simulink model "Supply_Chain_II"  (R2018b)
settings: Solver=VariableStepAuto  StartTime=0.0  StopTime=n_T  RelTol=1e-3
undefined symbols (not defined in the file or in its folder): D, m, MTBF_h, n, yoi
libraries: simulink x6
settings Model: Creator=Jorrit de Jong  LastModifiedBy=Jorrit de Jong

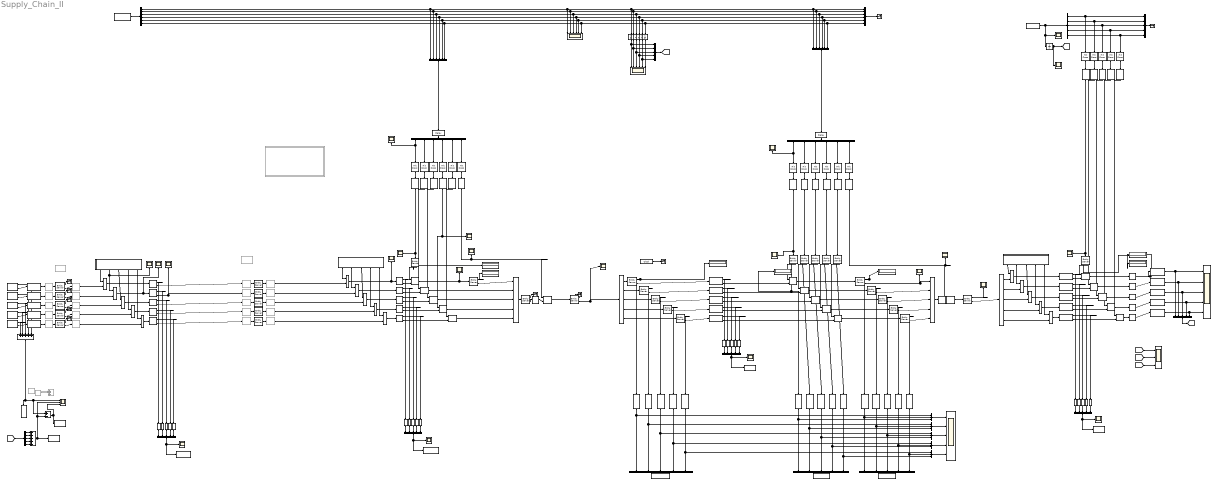
== system Supply_Chain_II ==
  note: DC
  note: Performance measurement JIT
  note: Local warehouse
  note: Island
  note: Performance measurement
  note: Terminal
  note: Performance measurement
  note: Control agent
  note: Performance measurement
  note: Control agent
  note: Source
  note: Performance measurement
  note: Scopes
  note: Nr of parts departed
  Add : Sum  Inputs=+++++
  Add1 : Sum  Inputs=+++++
  Add2 : Sum  Inputs=+-
  Add3 : Sum  Commented=on  Inputs=+++
  Arrived spares : Display
  Blade terminator : EntityTerminator  InputPortMessageModes=m  NumberEntitiesArrived=on
      settings: OutputPortMap=o0
  C terminator : EntityTerminator  InputPortMessageModes=m  NumberEntitiesArrived=on
      settings: OutputPortMap=o0
  Components arrived : Scope  NumInputPorts=5
  Constant : Constant  Commented=on  Value=5*20
  Constant1 : Constant  Commented=on  Value=5*20
  Counter : EntityServer  InputPortMessageModes=m  OutputPortMessageModes=n,m  Capacity=inf  ServiceTimeValue=0  NumberEntitiesDeparted=on
      settings: OutputPortMap=o0,o9
  Counter2 : EntityServer  InputPortMessageModes=m  OutputPortMessageModes=n,m  Capacity=inf  ServiceTimeValue=0  NumberEntitiesDeparted=on
      settings: OutputPortMap=o0,o9
  D terminator : EntityTerminator  InputPortMessageModes=m  NumberEntitiesArrived=on
      settings: OutputPortMap=o0
  DC transport signal : Scope
  DC trigger : Scope
  DC trigger system : Subsystem  Commented=on
  DC trigger1 : Scope
  Data Type Conversion{,1..39} (40 alike) : DataTypeConversion
  Demand - delivery flow : Scope  NumInputPorts=3
  Demux : Demux  Outputs=6
  Demux1 : Demux  Outputs=5
  Demux2 : Demux  Outputs=5
  Demux3 : Demux  Outputs=6
  Demux5 : Demux  Outputs=6
  Departed/Arrived components : Scope  NumInputPorts=3
  Digital Clock : DigitalClock
  Display : Display
  Display1 : Display
  Display2 : Display
  E terminator : EntityTerminator  InputPortMessageModes=m  NumberEntitiesArrived=on
      settings: OutputPortMap=o0
  Entity Input Switch : EntityInputSwitch  InputPortMessageModes=m,m,m,m,m  OutputPortMessageModes=m  NumberInputPorts=5
      settings: InputPortMap=u1,u2,u3,u4,u5
  Entity Input Switch{1..5,7..16} (15 alike) : EntityInputSwitch  InputPortMessageModes=m,m  OutputPortMessageModes=m
  Entity Input Switch6 : EntityInputSwitch  InputPortMessageModes=m,m,m,m,m  OutputPortMessageModes=m  NumberInputPorts=5
      settings: InputPortMap=u1,u2,u3,u4,u5
  Entity Output Switch : EntityOutputSwitch  InputPortMessageModes=m  OutputPortMessageModes=m,m,m,m,m  NumberOutputPorts=5  SwitchingCriterion=From attribute  SwitchAttributeName=PartNumber
      settings: OutputPortMap=o0,o1,o2,o3,o4
  Entity Output Switch1 : EntityOutputSwitch  InputPortMessageModes=m  OutputPortMessageModes=m,m,m,m,m  NumberOutputPorts=5  SwitchingCriterion=From attribute  SwitchAttributeName=PartNumber
      settings: OutputPortMap=o0,o1,o2,o3,o4
  Entity Gate{,1..16} (17 alike) : EntityGate  InputPortMessageModes=m,m  OutputPortMessageModes=m  OperatingMode=Release gate
  Entity Generator : EntityGenerator  OutputPortMessageModes=n,m  Period=MTBF_h(1,yoi)  GenerateEntityAtSimulationStart=off  AttributeName=PartNumber  NumberEntitiesDeparted=on  EntityType=Structured  EntityTypeName=Part
      settings: OutputPortMap=o0,o3
  Entity Generator1 : EntityGenerator  OutputPortMessageModes=n,m  Period=MTBF_h(2,yoi)  GenerateEntityAtSimulationStart=off  AttributeName=PartNumber  AttributeInitialValue=2  NumberEntitiesDeparted=on  EntityType=Structured  EntityTypeName=Part
      settings: OutputPortMap=o0,o3
  Entity Generator{5..16,18..22} (17 alike) : EntityGenerator  InputPortMessageModes=m  OutputPortMessageModes=m  GenerationMethod=Event-based  AttributeName=entity  AttributeInitialValue=0  EntityTypeName=Entity
      settings: InputPortMap=u0
  Entity Generator2 : EntityGenerator  OutputPortMessageModes=n,m  Period=MTBF_h(3,yoi)  GenerateEntityAtSimulationStart=off  AttributeName=PartNumber  AttributeInitialValue=3  NumberEntitiesDeparted=on  EntityType=Structured  EntityTypeName=Part
      settings: OutputPortMap=o0,o3
  Entity Generator3 : EntityGenerator  OutputPortMessageModes=n,m  Period=MTBF_h(4,yoi)  GenerateEntityAtSimulationStart=off  AttributeName=PartNumber  AttributeInitialValue=4  NumberEntitiesDeparted=on  EntityType=Structured  EntityTypeName=Part
      settings: OutputPortMap=o0,o3
  Entity Generator4 : EntityGenerator  OutputPortMessageModes=n,m  Period=MTBF_h(5,yoi)  GenerateEntityAtSimulationStart=off  AttributeName=PartNumber  AttributeInitialValue=5  NumberEntitiesDeparted=on  EntityType=Structured  EntityTypeName=Part
      settings: OutputPortMap=o0,o3
  Entity Queue{,1..4} (5 alike) : EntityQueue  InputPortMessageModes=m  OutputPortMessageModes=n,m  Capacity=20  NumberEntitiesInBlock=on
      settings: OutputPortMap=o1,o5
  Entity Queue{10..14} (5 alike) : EntityQueue  InputPortMessageModes=m  OutputPortMessageModes=m
      settings: OutputPortMap=o5
  Entity Queue{5..9} (5 alike) : EntityQueue  InputPortMessageModes=m  OutputPortMessageModes=n,m  NumberEntitiesInBlock=on
      settings: OutputPortMap=o1,o5
  Entity Server{,1..3,9..20} (16 alike) : EntityServer  InputPortMessageModes=m  OutputPortMessageModes=n,m  Capacity=inf  ServiceTimeValue=0  NumberEntitiesDeparted=on
      settings: OutputPortMap=o0,o9
  Entity Server{26..30} (5 alike) : EntityServer  InputPortMessageModes=m  OutputPortMessageModes=m  Capacity=inf  ServiceTimeSource=MATLAB action  ServiceTimeValue=D(2,3)  ServiceTimeAction=dt = normrnd(D(2,3),ts_sigma_distance(2,3));
  Entity Server{4..8} (5 alike) : EntityServer  InputPortMessageModes=m  OutputPortMessageModes=n,m  Capacity=inf  ServiceTimeSource=MATLAB action  ServiceTimeValue=D(1,2)  ServiceTimeAction=dt = normrnd(D(1,2),ts_sigma_distance(1,2));  NumberEntitiesDeparted=on
      settings: OutputPortMap=o0,o9
  Entity Store{,1..4,7..11} (10 alike) : EntityStore  InputPortMessageModes=m  OutputPortMessageModes=n,m  Capacity=20  NumberEntitiesInBlock=on
      settings: OutputPortMap=o1,o4
  Entity Store5 : EntityStore  InputPortMessageModes=m  OutputPortMessageModes=m  Capacity=inf
      settings: OutputPortMap=o4
  Entity Store6 : EntityStore  InputPortMessageModes=m  OutputPortMessageModes=m  Capacity=inf
      settings: OutputPortMap=o4
  Failures : Display
  Failures cumulated : Scope
  Failures3 : Display
  From Workspace : FromWorkspace  VariableName=Failure_events  SampleTime=0
  From Workspace1 : FromWorkspace  VariableName=Schedule_data  SampleTime=0
  Gearbox terminator : EntityTerminator  InputPortMessageModes=m  NumberEntitiesArrived=on
      settings: OutputPortMap=o0
  Hit Crossing{1..17} (17 alike) : HitCross  OutputPortMessageModes=m  HitCrossingDirection=rising  HitCrossingOutputType=Message
  Ini supply creator : Subsystem
  Ini supply creator1 : Subsystem
  Ini supply creator2 : Subsystem
  Integrator{,3..8} (7 alike) : Integrator
  Inventory level distribution center : Scope
  Inventory level island : Scope
  Inventory level local warehouse : Scope
  Inventory level terminal : Scope
  JIT Scope : Scope  NumInputPorts=5
  Loading : EntityServer  InputPortMessageModes=m  OutputPortMessageModes=n,m  Capacity=inf  ServiceTimeValue=1  NumberEntitiesDeparted=on
      settings: OutputPortMap=o0,o9
  Mux : Mux  Inputs=6
  Mux{1,4..9,15..17} (10 alike) : Mux  Inputs=5
  Mux10 : Mux  Inputs=6
  Mux{3,11..14} (5 alike) : Mux  Inputs=3
  Mux2 : Mux  Inputs=6
  Overall DC releaser : Scope
  Passed components : Display
  Post DC trigger : Scope
  Pre DC storage{,1..3} (4 alike) : Scope
  Resource Acquirer{,1..4} (5 alike) : EntityResourceAcquirer  Commented=through  InputPortMessageModes=m  OutputPortMessageModes=m  ResourceName=SD_Truck
      settings: OutputPortMap=o3
  Resource Acquirer{5..9} (5 alike) : EntityResourceAcquirer  Commented=through  InputPortMessageModes=m  OutputPortMessageModes=m  ResourceName=LD_trucks
      settings: OutputPortMap=o3
  Resource Releaser{,1..4} (5 alike) : EntityResourceReleaser  Commented=through  InputPortMessageModes=m  OutputPortMessageModes=m  ResourceToRelease=Selected  ResourceName=SD_Truck
  Resource Releaser{5..9} (5 alike) : EntityResourceReleaser  Commented=through  InputPortMessageModes=m  OutputPortMessageModes=m  ResourceToRelease=Selected  ResourceName=LD_trucks
  Resource Pool : EntityResourcePool  Commented=on  ResourceName=SD_Truck  ResourceAmount=30
  Resource Pool1 : EntityResourcePool  Commented=on  ResourceName=LD_trucks  ResourceAmount=20
  Road transport : EntityServer  InputPortMessageModes=m  OutputPortMessageModes=n,m  Capacity=inf  ServiceTimeSource=MATLAB action  ServiceTimeValue=20  ServiceTimeAction=dt = normrnd(D(3,4),ts_sigma_distance(3,4));  NumberEntitiesDeparted=on
      settings: OutputPortMap=o0,o9
  Road transport troughput : Scope
  Schedule data : Scope  NumInputPorts=6
  Schedule data accumulated : Scope  NumInputPorts=6
  Scope1 : Scope
  Scope4 : Scope
  Sea Transport : EntityServer  InputPortMessageModes=m  OutputPortMessageModes=n,m  Capacity=inf  ServiceTimeSource=MATLAB action  ServiceTimeValue=50  ServiceTimeAction=dt = normrnd(ts_vessel,2);  NumberEntitiesDeparted=on
      settings: OutputPortMap=o0,o9
  Sea transport post releaser : Scope
  Sea transport releaser : Scope
  Sea transport signal : Scope
  Sea transport sope : Scope
  Sea transport trigger : Scope
  Switched transport delay for linearization : TransportDelay  DelayTime=10  PadeOrder=1
  Switched transport delay for linearization1 : TransportDelay  PadeOrder=1
  Terminator{,1..9} (10 alike) : Terminator
  To Workspace : ToWorkspace  VariableName=inventory_level_island
      settings: Save2DSignal=2-D array (concatenate along first dimension)
  To Workspace1 : ToWorkspace  VariableName=com_caller
      settings: Save2DSignal=2-D array (concatenate along first dimension)
  To Workspace2 : ToWorkspace  VariableName=com_released
      settings: Save2DSignal=2-D array (concatenate along first dimension)
  To Workspace3 : ToWorkspace  VariableName=com_arrivals
      settings: Save2DSignal=2-D array (concatenate along first dimension)
  To Workspace4 : ToWorkspace  VariableName=inventory_level_terminal
      settings: Save2DSignal=2-D array (concatenate along first dimension)
  To Workspace5 : ToWorkspace  VariableName=inventory_level_LW
      settings: Save2DSignal=2-D array (concatenate along first dimension)
  To Workspace6 : ToWorkspace  VariableName=inventory_level_DC
      settings: Save2DSignal=2-D array (concatenate along first dimension)
  To Workspace7 : ToWorkspace  VariableName=departed_comps
      settings: Save2DSignal=2-D array (concatenate along first dimension)
  To Workspace8 : ToWorkspace  VariableName=arrived_comps
      settings: Save2DSignal=2-D array (concatenate along first dimension)
  To Workspace9 : ToWorkspace  VariableName=n_comps_in_sc
      settings: Save2DSignal=2-D array (concatenate along first dimension)
  wires:
  Mux12/1 -> JIT Scope/3  "Generators"
  Entity Queue2/1 -> Data Type Conversion5/1
  Entity Generator2/2 -> Entity Queue12/1
  Entity Gate9/1 -> Entity Input Switch/5
  Entity Input Switch7/1 -> Pre DC storage/1, Entity Store/1
  Entity Input Switch6/1 -> Entity Store6/1
  Switched transport delay for linearization1/1 -> Demux3/1
  Mux13/1 -> JIT Scope/4  "Rotor hubs"
  Data Type Conversion13/1 -> Mux6/3  "Generators"
  Counter2/2 -> Entity Gate5/1
  Demux3/1 -> Hit Crossing6/1, DC transport signal/1
  Entity Gate14/1 -> Entity Server15/1
  Mux8/1 -> To Workspace2/1
  Entity Generator3/2 -> Entity Queue13/1
  Entity Gate15/1 -> Entity Server16/1
  Entity Gate11/1 -> Entity Server/1
  Data Type Conversion/1 -> Mux3/3, Mux7/1  "Caller"
  Counter/2 -> Entity Input Switch/1
  Entity Output Switch1/1 -> Entity Server3/1
  Entity Generator6/1 -> Entity Server17/1
  Entity Store6/1 -> Entity Gate16/2
  Demux5/6 -> Hit Crossing2/1
  Loading/2 -> Entity Store5/1
  Demux1/1 -> Mux1/1, Hit Crossing13/1  "A"
  Entity Generator/2 -> Entity Queue10/1
  Ini supply creator/1(A) -> Entity Input Switch1/1
  Road transport/2 -> Entity Output Switch1/1, Road transport troughput/1
  Entity Gate12/1 -> Entity Server13/1
  Entity Generator11/1 -> DC trigger/1, Counter2/1
  Data Type Conversion20/1 -> Mux13/1, Mux9/4  "Arrivals"
  Demux5/1 -> Hit Crossing3/1, Sea transport signal/1
  Switched transport delay for linearization/1 -> Demux5/1
  Entity Input Switch1/1 -> Entity Queue/1
  Entity Generator1/2 -> Entity Queue11/1
  Demux5/5 -> Hit Crossing1/1
  Demux5/2 -> Hit Crossing4/1
  Entity Server11/1 -> Data Type Conversion20/1
  Entity Server10/2 -> Entity Queue7/1
  Data Type Conversion2/1 -> Mux3/1, Mux9/1  "Arrivals"
  Entity Generator8/1 -> Entity Server19/1
  Sea Transport/2 -> Entity Output Switch/1
  Data Type Conversion18/1 -> Mux11/1, Mux9/2  "Arrivals"
  Entity Output Switch1/4 -> Entity Server11/1
  Data Type Conversion24/1 -> Mux13/2, Mux8/4  "Released"
  Entity Server17/1 -> Data Type Conversion26/1
  Demux5/4 -> Hit Crossing12/1
  Entity Gate13/1 -> Entity Server14/1
  Entity Store2/2 -> Entity Gate7/2
  Data Type Conversion22/1 -> Mux11/2, Mux8/2  "Released"
  Entity Server19/1 -> Data Type Conversion28/1
  Entity Server18/1 -> Data Type Conversion27/1
  Data Type Conversion23/1 -> Mux8/3, Mux12/2  "Released"
  Mux1/1 -> Terminator2/1
  Data Type Conversion28/1 -> Mux13/3, Mux7/4  "Caller"
  Entity Gate/1 -> Blade terminator/1
  Entity Input Switch9/1 -> Entity Store2/1
  Data Type Conversion19/1 -> Mux12/1, Mux9/3  "Arrivals"
  Data Type Conversion7/1 -> Mux4/5  "Transformers"
  Entity Store2/1 -> Data Type Conversion13/1
  Entity Store1/1 -> Data Type Conversion17/1
  Demux3/5 -> Hit Crossing10/1
  Demux3/4 -> Hit Crossing9/1
  Demux3/3 -> Hit Crossing8/1
  Ini supply creator1/4(D) -> Entity Input Switch10/1
  Data Type Conversion8/1 -> Mux5/1  "Blades"
  Entity Generator20/1 -> Entity Gate2/1
  Entity Server16/1 -> Data Type Conversion25/1
  Entity Gate1/1 -> Gearbox terminator/1
  Ini supply creator1/2(B) -> Entity Input Switch8/1
  Entity Generator7/1 -> Entity Server18/1
  Demux5/3 -> Hit Crossing5/1
  Data Type Conversion21/1 -> Mux9/5, Mux14/1  "Arrivals"
  Entity Server16/2 -> Entity Input Switch6/5
  Demux3/6 -> Hit Crossing11/1
  Entity Store4/1 -> Data Type Conversion15/1
  Data Type Conversion27/1 -> Mux12/3, Mux7/3  "Caller"
  Entity Queue/1 -> Data Type Conversion3/1
  Data Type Conversion29/1 -> Mux7/5, Mux14/3  "Caller"
  Entity Store3/2 -> Entity Gate8/2
  Entity Output Switch/1 -> Entity Input Switch1/2
  Entity Generator15/1 -> Entity Gate9/1
  Entity Queue3/1 -> Data Type Conversion6/1
  Entity Gate4/1 -> E terminator/1
  Entity Store/2 -> Entity Gate5/2
  Entity Server3/1 -> Data Type Conversion2/1, Display2/1
  Mux7/1 -> To Workspace1/1
  Entity Server/1 -> Display/1, Data Type Conversion1/1
  Data Type Conversion14/1 -> Mux6/4  "Rotorhubs"
  Entity Server10/1 -> Data Type Conversion19/1
  Entity Server3/2 -> Entity Queue5/1
  Entity Server2/1 -> Display1/1, Data Type Conversion/1
  Entity Input Switch5/1 -> Entity Queue4/1
  Entity Queue5/1 -> Data Type Conversion8/1
  Entity Server2/2 -> Entity Gate11/1
  Entity Gate5/1 -> Post DC trigger/1, Counter/1
  Entity Generator10/1 -> Sea transport releaser/1, Entity Gate16/1
  Mux10/1 -> Switched transport delay for linearization1/1
  Entity Server1/2 -> Entity Gate/1
  Mux3/1 -> JIT Scope/1  "Blades"
  Mux2/1 -> Switched transport delay for linearization/1
  Entity Input Switch4/1 -> Entity Queue3/1
  Mux11/1 -> JIT Scope/2  "Gearboxes"
  Entity Input Switch2/1 -> Entity Queue1/1
  Entity Queue3/2 -> Entity Gate3/2
  From Workspace1/1 -> Demux/1
  Entity Queue6/2 -> Entity Gate12/2
  Entity Queue8/2 -> Entity Gate14/2
  Digital Clock/1 -> Terminator1/1
  Ini supply creator/4(D) -> Entity Input Switch4/1
  Entity Gate16/1 -> Sea Transport/1
  Blade terminator/1 -> Arrived spares/1, Data Type Conversion35/1
  Integrator/1 -> [Fail_comps], Failures cumulated/1
  Entity Output Switch/4 -> Entity Input Switch4/2
  Data Type Conversion25/1 -> Mux8/5, Mux14/2  "Released"
  Entity Generator14/1 -> Entity Gate8/1, DC trigger1/1
  Ini supply creator/3(C) -> Entity Input Switch3/1
  Sea Transport/1 -> Sea transport sope/1
  Entity Generator16/1 -> Entity Gate10/1, Overall DC releaser/1
  Ini supply creator/5(E) -> Entity Input Switch5/1
  Demux3/2 -> Hit Crossing7/1
  Counter2/1 -> Failures3/1
  Entity Store5/1 -> Entity Gate10/2
  Ini supply creator/2(B) -> Entity Input Switch2/1
  Ini supply creator1/5(E) -> Entity Input Switch11/1
  Entity Generator18/1 -> Entity Server1/1, Scope1/1
  Entity Generator12/1 -> Entity Gate6/1
  Mux9/1 -> To Workspace3/1
  Entity Gate2/1 -> C terminator/1
  Entity Queue1/2 -> Entity Gate1/2
  Entity Queue/2 -> Entity Gate/2
  Entity Generator22/1 -> Entity Gate4/1
  Entity Input Switch/1 -> Loading/1
  Entity Gate8/1 -> Entity Input Switch/4
  Demux1/3 -> Mux1/3, Hit Crossing15/1  "C"
  Entity Queue2/2 -> Entity Gate2/2
  Entity Server1/1 -> Failures/1
  Entity Gate7/1 -> Entity Input Switch/3
  Data Type Conversion26/1 -> Mux11/3, Mux7/2  "Caller"
  Entity Server19/2 -> Entity Gate14/1
  Entity Server/2 -> Sea transport post releaser/1, Entity Input Switch6/1
  Entity Server13/1 -> Data Type Conversion22/1
  Entity Server20/2 -> Entity Gate15/1
  Entity Input Switch10/1 -> Entity Store3/1
  Counter/1 -> Passed components/1
  Mux/1 -> Terminator4/1
  Entity Output Switch1/3 -> Entity Server10/1
  Entity Server9/1 -> Data Type Conversion18/1
  Entity Server12/2 -> Entity Queue9/1
  Entity Server14/2 -> Entity Input Switch6/3
  Entity Server12/1 -> Data Type Conversion21/1
  Entity Gate10/1 -> Road transport/1
  Entity Server13/2 -> Entity Input Switch6/2
  Entity Server15/2 -> Entity Input Switch6/4
  Entity Queue9/2 -> Entity Gate15/2
  Entity Generator5/1 -> Entity Server2/1, Sea transport trigger/1
  Demux1/4 -> Mux1/4, Hit Crossing16/1  "D"
  Data Type Conversion12/1 -> Mux5/5  "Transformers"
  Data Type Conversion11/1 -> Mux5/4  "Rotorhubs"
  Entity Queue5/2 -> Entity Gate11/2
  Entity Generator19/1 -> Entity Gate1/1
  Entity Server17/2 -> Entity Gate12/1
  Ini supply creator1/3(C) -> Entity Input Switch9/1
  Entity Input Switch8/1 -> Entity Store1/1
  Entity Output Switch1/2 -> Entity Server9/1
  Ini supply creator1/1(A) -> Entity Input Switch7/1
  Demux1/5 -> Mux1/5, Hit Crossing17/1  "E"
  Entity Server11/2 -> Entity Queue8/1
  Data Type Conversion1/1 -> Mux3/2, Mux8/1  "Released"
  Entity Queue7/2 -> Entity Gate13/2
  Mux14/1 -> JIT Scope/5  "Transformer"
  Entity Store1/2 -> Entity Gate6/2
  Entity Store/1 -> Data Type Conversion16/1
  Demux1/2 -> Mux1/2, Hit Crossing14/1  "B"
  Data Type Conversion15/1 -> Mux6/5  "Transformers"
  Data Type Conversion17/1 -> Mux6/2  "Gearboxes"
  Entity Output Switch/2 -> Entity Input Switch2/2
  Entity Generator13/1 -> Entity Gate7/1
  Entity Input Switch11/1 -> Entity Store4/1
  Data Type Conversion16/1 -> Mux6/1  "Blades"
  Entity Server15/1 -> Data Type Conversion24/1
  Entity Queue7/1 -> Data Type Conversion10/1
  Entity Queue4/2 -> Entity Gate4/2
  Data Type Conversion5/1 -> Mux4/3  "Generators"
  Entity Queue1/1 -> Data Type Conversion4/1
  Entity Queue9/1 -> Data Type Conversion12/1
  Entity Server9/2 -> Entity Queue6/1
  Entity Store3/1 -> Data Type Conversion14/1
  From Workspace/1 -> Integrator/1, Scope4/1, Demux1/1
  Mux5/1 -> To Workspace4/1, Inventory level terminal/1
  Entity Output Switch/3 -> Entity Input Switch3/2
  Entity Server20/1 -> Data Type Conversion29/1
  Entity Queue6/1 -> Data Type Conversion9/1
  Entity Output Switch1/5 -> Entity Server12/1
  Entity Server18/2 -> Entity Gate13/1
  Data Type Conversion9/1 -> Mux5/2  "Gearboxes"
  Data Type Conversion6/1 -> Mux4/4  "Rotorhubs"
  Entity Generator21/1 -> Entity Gate3/1
  Data Type Conversion10/1 -> Mux5/3  "Generators"
  Mux6/1 -> To Workspace5/1, Inventory level local warehouse/1
  Entity Queue4/1 -> Data Type Conversion7/1
  Data Type Conversion4/1 -> Mux4/2  "Gearboxes"
  Entity Queue8/1 -> Data Type Conversion11/1
  Entity Output Switch/5 -> Entity Input Switch5/2
  Data Type Conversion3/1 -> Mux4/1  "Blades"
  Entity Generator9/1 -> Entity Server20/1
  Entity Gate6/1 -> Entity Input Switch/2
  Entity Input Switch3/1 -> Entity Queue2/1
  Entity Server14/1 -> Data Type Conversion23/1
  Entity Gate3/1 -> D terminator/1
  Entity Generator4/2 -> Entity Queue14/1
  Mux4/1 -> To Workspace/1, Inventory level island/1
  Entity Store4/2 -> Entity Gate9/2
  Entity Store11/2 -> Resource Acquirer4/1
  Entity Store10/2 -> Resource Acquirer3/1
  Entity Store9/2 -> Resource Acquirer2/1
  Entity Store8/2 -> Resource Acquirer1/1, Pre DC storage3/1
  Entity Store7/2 -> Resource Acquirer/1
  Resource Acquirer/1 -> Entity Server26/1
  Resource Releaser/1 -> Entity Input Switch7/2
  Resource Acquirer1/1 -> Entity Server27/1
  Resource Acquirer2/1 -> Entity Server28/1
  Resource Acquirer3/1 -> Entity Server29/1
  Resource Acquirer4/1 -> Entity Server30/1
  Resource Releaser1/1 -> Entity Input Switch8/2
  Resource Releaser2/1 -> Entity Input Switch9/2
  Resource Releaser3/1 -> Entity Input Switch10/2
  Resource Releaser4/1 -> Entity Input Switch11/2
  Entity Server26/1 -> Resource Releaser/1
  Entity Server27/1 -> Resource Releaser1/1
  Entity Server28/1 -> Resource Releaser2/1
  Entity Server29/1 -> Resource Releaser3/1
  Entity Server30/1 -> Resource Releaser4/1
  Data Type Conversion32/1 -> Mux15/5  "Transformers"
  Data Type Conversion34/1 -> Mux15/2  "Gearboxes"
  Data Type Conversion33/1 -> Mux15/1  "Blades"
  Entity Store11/1 -> Data Type Conversion32/1
  Entity Store8/1 -> Data Type Conversion34/1
  Entity Store9/1 -> Data Type Conversion30/1
  Entity Store10/1 -> Data Type Conversion31/1
  Entity Store7/1 -> Data Type Conversion33/1
  Data Type Conversion30/1 -> Mux15/3  "Generators"
  Mux15/1 -> To Workspace6/1, Inventory level distribution center/1
  Data Type Conversion31/1 -> Mux15/4  "Rotorhubs"
  Entity Server4/1 -> Terminator/1
  Entity Server5/1 -> Terminator3/1
  Entity Server6/1 -> Terminator5/1
  Entity Server7/1 -> Terminator6/1
  Entity Server8/1 -> Terminator7/1
  Hit Crossing6/1 -> Entity Generator11/1
  Hit Crossing11/1 -> Entity Generator16/1
  Hit Crossing8/1 -> Entity Generator13/1
  Hit Crossing7/1 -> Entity Generator12/1
  Hit Crossing10/1 -> Entity Generator15/1
  Hit Crossing9/1 -> Entity Generator14/1
  Hit Crossing3/1 -> Entity Generator5/1
  Hit Crossing2/1 -> Entity Generator10/1
  Hit Crossing5/1 -> Entity Generator7/1
  Hit Crossing4/1 -> Entity Generator6/1
  Hit Crossing1/1 -> Entity Generator9/1
  Hit Crossing12/1 -> Entity Generator8/1
  Hit Crossing14/1 -> Entity Generator19/1
  Hit Crossing16/1 -> Entity Generator21/1
  Hit Crossing13/1 -> Entity Generator18/1
  Hit Crossing15/1 -> Entity Generator20/1
  Hit Crossing17/1 -> Entity Generator22/1
  Mux16/1 -> [Arr_comps]
  Data Type Conversion38/1 -> Mux16/4, Components arrived/4
  Data Type Conversion36/1 -> Mux16/2, Components arrived/2
  Data Type Conversion37/1 -> Mux16/3, Components arrived/3
  Data Type Conversion39/1 -> Mux16/5, Components arrived/5
  Data Type Conversion35/1 -> Mux16/1, Components arrived/1
  Gearbox terminator/1 -> Data Type Conversion36/1
  C terminator/1 -> Data Type Conversion37/1
  D terminator/1 -> Data Type Conversion38/1
  E terminator/1 -> Data Type Conversion39/1
  [Fail_comps] -> Demand - delivery flow/1  "Failures"
  [Arr_comps] -> Demand - delivery flow/3  "Delivered"
  [Sche_comps] -> Demand - delivery flow/2  "Scheduled"
  Add2/1 -> To Workspace9/1, Departed/Arrived components/3  "Result"
  Add1/1 -> To Workspace8/1, Departed/Arrived components/2, Add2/2  "Arrivals"
  Demux2/5 -> Add1/5
  Demux2/1 -> Add1/1
  Demux2/2 -> Add1/2
  [Arr_comps] -> Demux2/1  "Delivered"
  Constant1/1 -> Add3/2
  Demux2/3 -> Add1/3
  Constant/1 -> Add3/1
  Entity Generator1/1 -> Add/4
  Entity Generator/1 -> Add/5
  Entity Generator3/1 -> Add/2
  Demux2/4 -> Add1/4
  Add/1 -> To Workspace7/1, Add2/1, Departed/Arrived components/1  "Departs"
  Entity Generator2/1 -> Add/3
  Entity Generator4/1 -> Add/1
  Demux/6 -> Schedule data/6, Integrator8/1, Mux2/6, Mux/6, Mux10/6  "t"
  Integrator3/1 -> Mux17/1, Schedule data accumulated/1
  Demux/4 -> Schedule data/4, Integrator6/1, Mux2/4, Mux/4, Mux10/4  "D"
  Integrator8/1 -> Schedule data accumulated/6
  Demux/3 -> Schedule data/3, Integrator5/1, Mux2/3, Mux/3, Mux10/3  "C"
  Demux/2 -> Schedule data/2, Integrator4/1, Mux2/2, Mux/2, Mux10/2  "B"
  Demux/1 -> Schedule data/1, Integrator3/1, Mux2/1, Mux/1, Mux10/1  "A"
  Integrator5/1 -> Mux17/3, Schedule data accumulated/3
  Integrator7/1 -> Mux17/5, Schedule data accumulated/5
  Integrator4/1 -> Mux17/2, Schedule data accumulated/2
  Integrator6/1 -> Mux17/4, Schedule data accumulated/4
  Mux17/1 -> [Sche_comps]
  Demux/5 -> Schedule data/5, Integrator7/1, Mux2/5, Mux/5, Mux10/5  "E"
  Ini supply creator2/2(B) -> Pre DC storage1/1, Entity Input Switch15/1
  Ini supply creator2/5(E) -> Entity Input Switch13/1
  Ini supply creator2/1(A) -> Entity Input Switch14/1
  Ini supply creator2/3(C) -> Entity Input Switch16/1
  Ini supply creator2/4(D) -> Entity Input Switch12/1
  Entity Server4/2 -> Resource Releaser5/1
  Entity Server5/2 -> Resource Releaser6/1
  Entity Server6/2 -> Resource Releaser7/1
  Entity Server7/2 -> Resource Releaser8/1
  Entity Server8/2 -> Resource Releaser9/1
  Entity Input Switch14/1 -> Entity Store7/1
  Entity Input Switch15/1 -> Pre DC storage2/1, Entity Store8/1
  Entity Input Switch16/1 -> Entity Store9/1
  Entity Input Switch12/1 -> Entity Store10/1
  Entity Input Switch13/1 -> Entity Store11/1
  Resource Acquirer9/1 -> Entity Server8/1
  Resource Acquirer8/1 -> Entity Server7/1
  Resource Acquirer5/1 -> Entity Server4/1
  Resource Acquirer6/1 -> Entity Server5/1
  Resource Acquirer7/1 -> Entity Server6/1
  Resource Releaser9/1 -> Entity Input Switch13/2
  Resource Releaser5/1 -> Entity Input Switch14/2
  Resource Releaser7/1 -> Entity Input Switch16/2
  Resource Releaser8/1 -> Entity Input Switch12/2
  Resource Releaser6/1 -> Entity Input Switch15/2
  Road transport/1 -> Terminator8/1
  Loading/1 -> Terminator9/1
  Entity Queue10/1 -> Resource Acquirer5/1
  Entity Queue11/1 -> Resource Acquirer6/1
  Entity Queue12/1 -> Resource Acquirer7/1
  Entity Queue13/1 -> Resource Acquirer8/1
  Entity Queue14/1 -> Resource Acquirer9/1

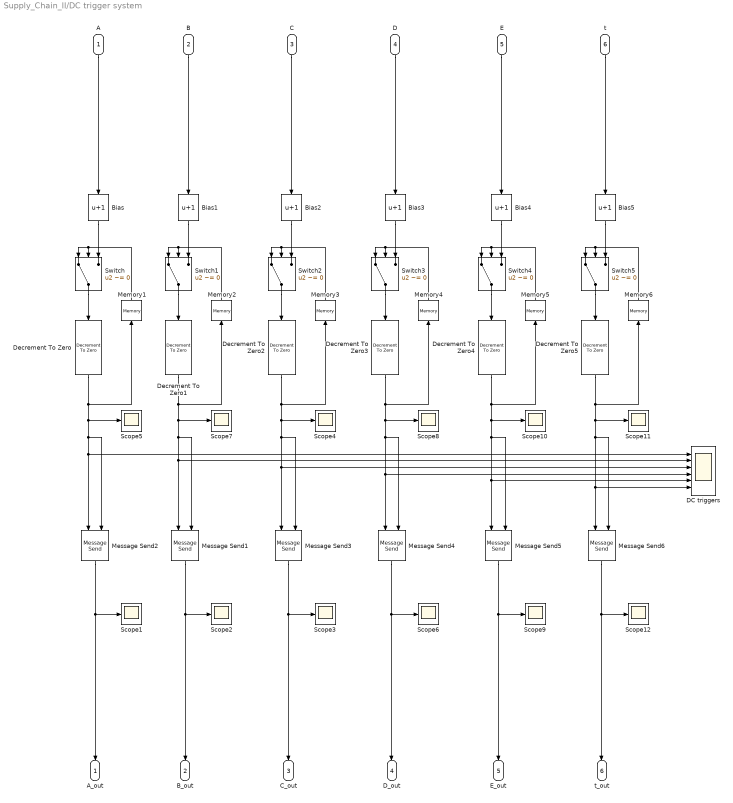
== system Supply_Chain_II/DC trigger system ==
  A : Inport
  B : Inport  Port=2
  C : Inport  Port=3
  D : Inport  Port=4
  E : Inport  Port=5
  t : Inport  Port=6
  Bias{,1..5} (6 alike) : Bias  Bias=1
  DC triggers : Scope  NumInputPorts=6
  Decrement To Zero{,1..5} (6 alike) : simulink/Additional Math & Discrete/Additional Math: Increment - Decrement/Decrement To Zero
      settings: SourceProductName=Simulink  SourceProductBaseCode=SL
  Memory{1..6} (6 alike) : Memory
  Message Send{1..6} (6 alike) : MessageSend  OutputPortMessageModes=m  ShowEnablePort=on
      settings: InputPortMap=e0,u1
  Scope{1..12} (12 alike) : Scope
  Switch{,1..5} (6 alike) : Switch  Criteria=u2 ~= 0
  A_out : Outport
  B_out : Outport  Port=2
  C_out : Outport  Port=3
  D_out : Outport  Port=4
  E_out : Outport  Port=5
  t_out : Outport  Port=6
  wires:
  Bias1/1 -> Switch1/3
  Decrement To Zero/1 -> Message Send2/1, DC triggers/1, Message Send2/2, Scope5/1, Memory1/1
  Switch/1 -> Decrement To Zero/1
  Decrement To Zero1/1 -> Message Send1/1, DC triggers/2, Message Send1/2, Scope7/1, Memory2/1
  Memory1/1 -> Switch/2, Switch/1
  Memory2/1 -> Switch1/2, Switch1/1
  Bias/1 -> Switch/3
  Message Send1/1 -> Scope2/1, B_out/1
  Switch1/1 -> Decrement To Zero1/1
  Message Send2/1 -> Scope1/1, A_out/1
  A/1 -> Bias/1
  B/1 -> Bias1/1
  Bias2/1 -> Switch2/3
  Message Send3/1 -> Scope3/1, C_out/1
  Memory3/1 -> Switch2/2, Switch2/1
  Switch2/1 -> Decrement To Zero2/1
  C/1 -> Bias2/1
  Decrement To Zero2/1 -> Message Send3/1, DC triggers/3, Message Send3/2, Scope4/1, Memory3/1
  Bias3/1 -> Switch3/3
  Message Send4/1 -> Scope6/1, D_out/1
  Memory4/1 -> Switch3/2, Switch3/1
  Switch3/1 -> Decrement To Zero3/1
  D/1 -> Bias3/1
  Decrement To Zero3/1 -> Message Send4/1, DC triggers/4, Message Send4/2, Scope8/1, Memory4/1
  Bias4/1 -> Switch4/3
  Message Send5/1 -> Scope9/1, E_out/1
  Memory5/1 -> Switch4/2, Switch4/1
  Switch4/1 -> Decrement To Zero4/1
  E/1 -> Bias4/1
  Decrement To Zero4/1 -> Message Send5/1, DC triggers/5, Message Send5/2, Scope10/1, Memory5/1
  Bias5/1 -> Switch5/3
  Message Send6/1 -> Scope12/1, t_out/1
  Decrement To Zero5/1 -> DC triggers/6, Message Send6/1, Message Send6/2, Scope11/1, Memory6/1
  Switch5/1 -> Decrement To Zero5/1
  Memory6/1 -> Switch5/2, Switch5/1
  t/1 -> Bias5/1

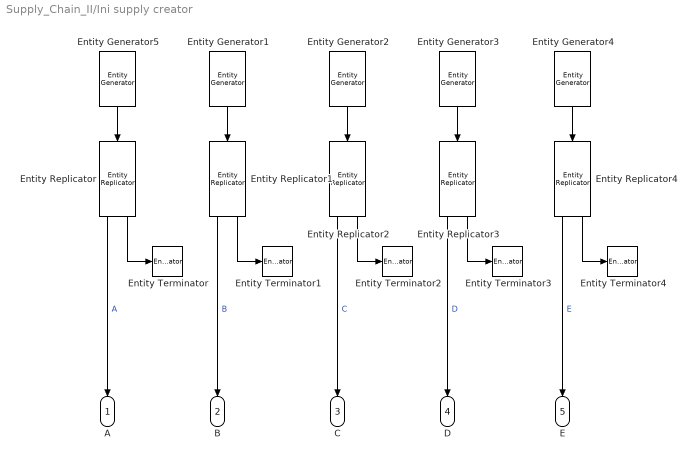
== system Supply_Chain_II/Ini supply creator ==
  Entity Generator1 : EntityGenerator  OutputPortMessageModes=m  Period=inf  AttributeName=PartNumber  AttributeInitialValue=2  EntityType=Structured  EntityTypeName=Part
  Entity Generator2 : EntityGenerator  OutputPortMessageModes=m  Period=inf  AttributeName=PartNumber  AttributeInitialValue=3  EntityType=Structured  EntityTypeName=Part
  Entity Generator3 : EntityGenerator  OutputPortMessageModes=m  Period=inf  AttributeName=PartNumber  AttributeInitialValue=4  EntityType=Structured  EntityTypeName=Part
  Entity Generator4 : EntityGenerator  OutputPortMessageModes=m  Period=inf  AttributeName=PartNumber  AttributeInitialValue=5  EntityType=Structured  EntityTypeName=Part
  Entity Generator5 : EntityGenerator  OutputPortMessageModes=m  Period=inf  AttributeName=PartNumber  EntityType=Structured  EntityTypeName=Part
  Entity Replicator{,1..4} (5 alike) : EntityReplicator  InputPortMessageModes=m  OutputPortMessageModes=m,m  ReplicasDepartFrom=Single output port  NumberReplicas=20
  Entity Terminator{,1..4} (5 alike) : EntityTerminator  InputPortMessageModes=m
  A : Outport
  B : Outport  Port=2
  C : Outport  Port=3
  D : Outport  Port=4
  E : Outport  Port=5
  wires:
  Entity Generator5/1 -> Entity Replicator/1
  Entity Replicator/2 -> Entity Terminator/1
  Entity Replicator/1 -> A/1  "A"
  Entity Replicator1/1 -> B/1  "B"
  Entity Generator1/1 -> Entity Replicator1/1
  Entity Replicator1/2 -> Entity Terminator1/1
  Entity Replicator2/1 -> C/1  "C"
  Entity Generator2/1 -> Entity Replicator2/1
  Entity Replicator2/2 -> Entity Terminator2/1
  Entity Replicator3/1 -> D/1  "D"
  Entity Generator3/1 -> Entity Replicator3/1
  Entity Replicator3/2 -> Entity Terminator3/1
  Entity Replicator4/1 -> E/1  "E"
  Entity Generator4/1 -> Entity Replicator4/1
  Entity Replicator4/2 -> Entity Terminator4/1

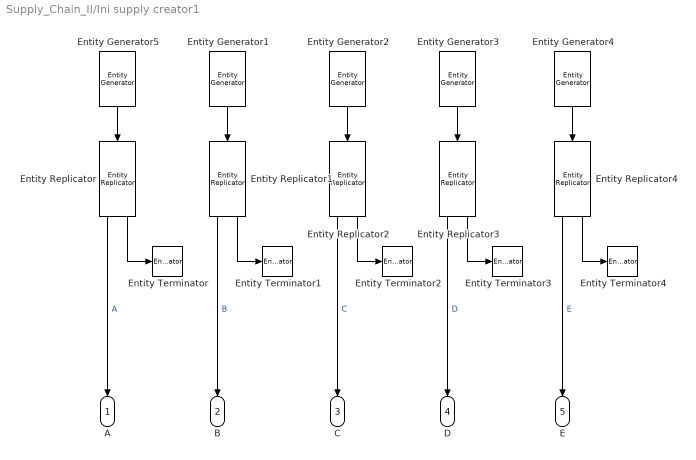
== system Supply_Chain_II/Ini supply creator1 ==
  Entity Generator1 : EntityGenerator  OutputPortMessageModes=m  Period=inf  AttributeName=PartNumber  AttributeInitialValue=2  EntityType=Structured  EntityTypeName=Part
  Entity Generator2 : EntityGenerator  OutputPortMessageModes=m  Period=inf  AttributeName=PartNumber  AttributeInitialValue=3  EntityType=Structured  EntityTypeName=Part
  Entity Generator3 : EntityGenerator  OutputPortMessageModes=m  Period=inf  AttributeName=PartNumber  AttributeInitialValue=4  EntityType=Structured  EntityTypeName=Part
  Entity Generator4 : EntityGenerator  OutputPortMessageModes=m  Period=inf  AttributeName=PartNumber  AttributeInitialValue=5  EntityType=Structured  EntityTypeName=Part
  Entity Generator5 : EntityGenerator  OutputPortMessageModes=m  Period=inf  AttributeName=PartNumber  EntityType=Structured  EntityTypeName=Part
  Entity Replicator{,1..4} (5 alike) : EntityReplicator  InputPortMessageModes=m  OutputPortMessageModes=m,m  ReplicasDepartFrom=Single output port  NumberReplicas=20
  Entity Terminator{,1..4} (5 alike) : EntityTerminator  InputPortMessageModes=m
  A : Outport
  B : Outport  Port=2
  C : Outport  Port=3
  D : Outport  Port=4
  E : Outport  Port=5
  wires:
  Entity Generator5/1 -> Entity Replicator/1
  Entity Replicator/2 -> Entity Terminator/1
  Entity Replicator/1 -> A/1  "A"
  Entity Replicator1/1 -> B/1  "B"
  Entity Generator1/1 -> Entity Replicator1/1
  Entity Replicator1/2 -> Entity Terminator1/1
  Entity Replicator2/1 -> C/1  "C"
  Entity Generator2/1 -> Entity Replicator2/1
  Entity Replicator2/2 -> Entity Terminator2/1
  Entity Replicator3/1 -> D/1  "D"
  Entity Generator3/1 -> Entity Replicator3/1
  Entity Replicator3/2 -> Entity Terminator3/1
  Entity Replicator4/1 -> E/1  "E"
  Entity Generator4/1 -> Entity Replicator4/1
  Entity Replicator4/2 -> Entity Terminator4/1

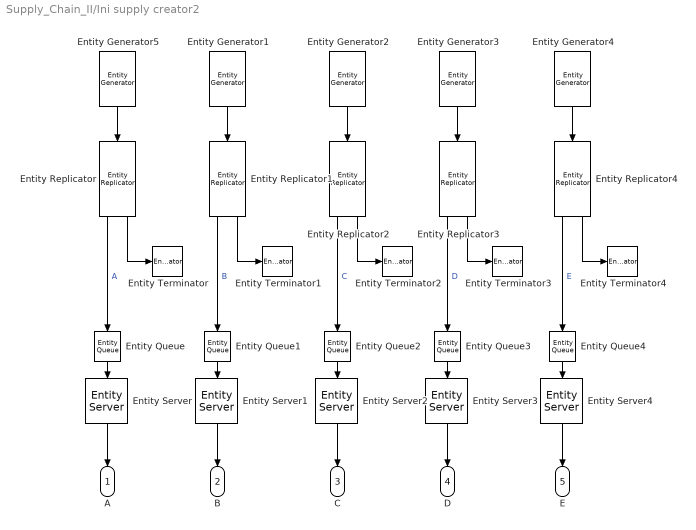
== system Supply_Chain_II/Ini supply creator2 ==
  Entity Generator1 : EntityGenerator  OutputPortMessageModes=m  Period=inf  AttributeName=PartNumber  AttributeInitialValue=2  EntityType=Structured  EntityTypeName=Part
  Entity Generator2 : EntityGenerator  OutputPortMessageModes=m  Period=inf  AttributeName=PartNumber  AttributeInitialValue=3  EntityType=Structured  EntityTypeName=Part
  Entity Generator3 : EntityGenerator  OutputPortMessageModes=m  Period=inf  AttributeName=PartNumber  AttributeInitialValue=4  EntityType=Structured  EntityTypeName=Part
  Entity Generator4 : EntityGenerator  OutputPortMessageModes=m  Period=inf  AttributeName=PartNumber  AttributeInitialValue=5  EntityType=Structured  EntityTypeName=Part
  Entity Generator5 : EntityGenerator  OutputPortMessageModes=m  Period=inf  AttributeName=PartNumber  EntityType=Structured  EntityTypeName=Part
  Entity Queue{,1..4} (5 alike) : EntityQueue  InputPortMessageModes=m  OutputPortMessageModes=m
      settings: OutputPortMap=o5
  Entity Replicator{,1..4} (5 alike) : EntityReplicator  InputPortMessageModes=m  OutputPortMessageModes=m,m  ReplicasDepartFrom=Single output port  NumberReplicas=20
  Entity Server{,1..4} (5 alike) : EntityServer  InputPortMessageModes=m  OutputPortMessageModes=m  Capacity=1  ServiceTimeValue=1
  Entity Terminator{,1..4} (5 alike) : EntityTerminator  InputPortMessageModes=m
  A : Outport
  B : Outport  Port=2
  C : Outport  Port=3
  D : Outport  Port=4
  E : Outport  Port=5
  wires:
  Entity Generator5/1 -> Entity Replicator/1
  Entity Replicator/2 -> Entity Terminator/1
  Entity Replicator/1 -> Entity Queue/1  "A"
  Entity Replicator1/1 -> Entity Queue1/1  "B"
  Entity Generator1/1 -> Entity Replicator1/1
  Entity Replicator1/2 -> Entity Terminator1/1
  Entity Replicator2/1 -> Entity Queue2/1  "C"
  Entity Generator2/1 -> Entity Replicator2/1
  Entity Replicator2/2 -> Entity Terminator2/1
  Entity Replicator3/1 -> Entity Queue3/1  "D"
  Entity Generator3/1 -> Entity Replicator3/1
  Entity Replicator3/2 -> Entity Terminator3/1
  Entity Replicator4/1 -> Entity Queue4/1  "E"
  Entity Generator4/1 -> Entity Replicator4/1
  Entity Replicator4/2 -> Entity Terminator4/1
  Entity Server/1 -> A/1
  Entity Queue/1 -> Entity Server/1
  Entity Queue1/1 -> Entity Server1/1
  Entity Server1/1 -> B/1
  Entity Queue2/1 -> Entity Server2/1
  Entity Server2/1 -> C/1
  Entity Queue3/1 -> Entity Server3/1
  Entity Server3/1 -> D/1
  Entity Queue4/1 -> Entity Server4/1
  Entity Server4/1 -> E/1
